simulink model "part2"  (R2018b)
settings: Solver=VariableStepAuto  StartTime=0.0  StopTime=10.0  RelTol=1e-3
settings Model: Creator=Tianshi_Fu  LastModifiedBy=Tianshi_Fu

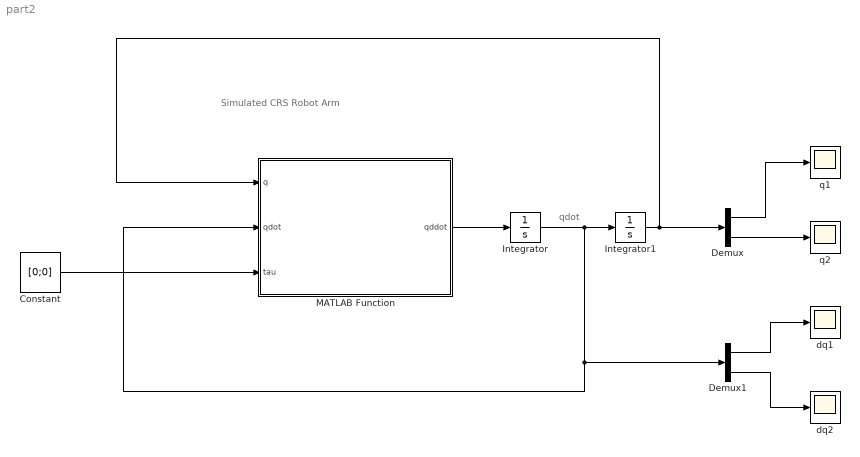
== system part2 ==
  note: qdot
  note: Simulated CRS Robot Arm
  Constant : Constant  Value=[0;0]
  Demux : Demux  Outputs=2
  Demux1 : Demux  Outputs=2
  Integrator : Integrator  InitialCondition=[0;0]
  Integrator1 : Integrator  InitialCondition=[pi/2;0]
  MATLAB Function : MATLAB Function  TreatAsAtomicUnit=on
  dq1 : Scope
  dq2 : Scope
  q1 : Scope
  q2 : Scope
  wires:
  Demux/2 -> q2/1
  Demux1/1 -> dq1/1
  Integrator/1 -> Demux1/1, MATLAB Function/2(qdot), Integrator1/1
  Demux/1 -> q1/1
  Integrator1/1 -> Demux/1, MATLAB Function/1(q)
  Demux1/2 -> dq2/1
  MATLAB Function/1(qddot) -> Integrator/1
  Constant/1 -> MATLAB Function/3(tau)

== matlab function part2/MATLAB Function ==
  data: q input; qddot output; qdot input; tau input
function qddot = fcn(q,qdot,tau)

p = [0.0300; 0.0128; 0.0076; 0.0753; 0.0298];
g = 9.805;


D = [p(1) -p(3)*sin(q(2)-q(1)); -p(3)*sin(q(2)-q(1)) p(2)];
C = [0 -p(3)*cos(q(2)-q(1))*qdot(2); p(3)*cos(q(2)-q(1))*qdot(1) 0];
G = [-p(4)*g*sin(q(1)); -p(5)*g*cos(q(2))];

qddot = inv(D)*tau - inv(D)*C*qdot - inv(D)*G;
